simulink model "SecRwRtStHdrstFwdBkwdCtrl"  (R2018b)
settings: Solver=FixedStepDiscrete  StartTime=0.0  StopTime=10.0  FixedStep=0.01  RelTol=1e-3
undefined symbols (not defined in the file or in its folder): KeSMSuMdMotFinshdTm_Val, KeSMSuMdRetryTm1_Val, KeSMSuModeReqDurgTm_Val, KeSMSwSecRwRtStHdrstFwdBkwdEnTrigBitMask_Val
libraries: StCtrlLib x1
settings Model: Creator=sn2xws  LastModifiedBy=sn2xws
settings DataIOCC: SaveFormat=StructureWithTime
settings OptimizationCC: DefaultParameterBehavior=Inlined  EnhancedBackFolding=on  PassReuseOutputArgsAs=Individual arguments  ZeroExternalMemoryAtStartup=off  ZeroInternalMemoryAtStartup=off  OptimizeBlockOrder=speed  DifferentSizesBufferReuse=on  OptimizationCustomize=off
settings DebuggingCC: ParameterTunabilityLossMsg=error
settings ModelReferenceCC: ModelReferenceNumInstancesAllowed=Single
settings SFSimCC: MATLABDynamicMemAlloc=off
settings RTWCC: SystemTargetFile=autosar.tlc  GenCodeOnly=on  TemplateMakefile=ert_default_tmf  Description=AUTOSAR  GenerateReport=on  IncludeHyperlinkInReport=on  LaunchReport=on  GenerateTraceInfo=on  GenerateTraceReport=on  GenerateTraceReportSl=on  GenerateTraceReportSf=on  GenerateTraceReportEml=on
settings CodeAppCC: ForceParamTrailComments=on  IgnoreCustomStorageClasses=off  OperatorAnnotations=on  SimulinkDataObjDesc=on  SFDataObjDesc=on  InsertBlockDesc=on
settings STFCustomTargetCC: TargetLangStandard=C99 (ISO)  MultiwordLength=256  ParMdlRefBuildCompliant=on  CompOptLevelCompliant=on  IncludeMdlTerminateFcn=off  CombineOutputUpdateFcns=on  SuppressErrorStatus=on  ERTCustomFileBanners=on  SupportNonFinite=off  SupportComplex=off  SupportContinuousTime=off  SupportNonInlinedSFcns=off  RemoveResetFunc=on  MATLABClassNameForMDSCustomization=Simulink.SoftwareTarget.ERTCustomization  AutosarCompliant=on  UseToolchainInfoCompliant=on  LookupTableObjectStructAxisOrder=2,1,3,4,...  LUTObjectStructOrderEvenSpacing=Size,Table,Breakpoints  SystemTargetFile=autosar.tlc
settings ERTTargetCC: TargetLangStandard=C99 (ISO)  ConcurrentExecutionCompliant=off  IncludeMdlTerminateFcn=off  SuppressErrorStatus=on  SupportNonFinite=off  SupportComplex=off  ModelStepFunctionPrototypeControlCompliant=off  CPPClassGenCompliant=off  AutosarCompliant=on  LookupTableObjectStructAxisOrder=2,1,3,4,...  LUTObjectStructOrderEvenSpacing=Size,Table,Breakpoints  InlinedParameterPlacement=NonHierarchical  ERTCustomFileTemplate=example_file_process.tlc  ERTFilePackagingFormat=Compact

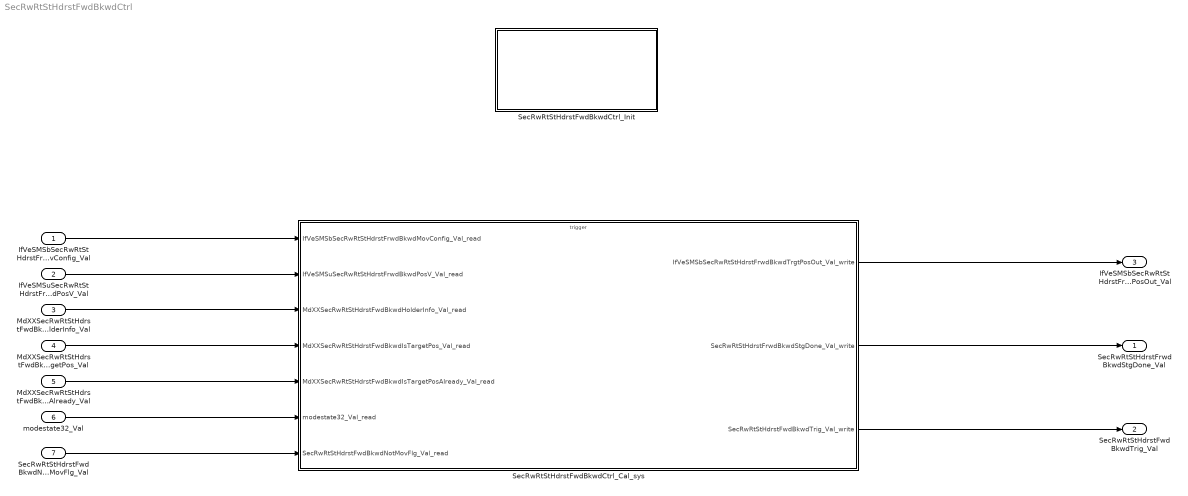
== system SecRwRtStHdrstFwdBkwdCtrl ==
  IfVeSMSbSecRwRtStHdrstFrwdBkwdMovConfig_Val : Inport  OutDataTypeStr=boolean  PortDimensions=1
  IfVeSMSuSecRwRtStHdrstFrwdBkwdPosV_Val : Inport  Port=2  OutDataTypeStr=boolean  PortDimensions=1
  MdXXSecRwRtStHdrstFwdBkwdHolderInfo_Val : Inport  Port=3  OutDataTypeStr=uint32  PortDimensions=1
  MdXXSecRwRtStHdrstFwdBkwdIsTargetPos_Val : Inport  Port=4  OutDataTypeStr=uint32  PortDimensions=1
  MdXXSecRwRtStHdrstFwdBkwdIsTargetPosAlready_Val : Inport  Port=5  OutDataTypeStr=uint32  PortDimensions=1
  modestate32_Val : Inport  Port=6  OutDataTypeStr=uint32  PortDimensions=1
  SecRwRtStHdrstFwdBkwdNotMovFlg_Val : Inport  Port=7  OutDataTypeStr=boolean  PortDimensions=1
  SecRwRtStHdrstFwdBkwdCtrl_Cal_sys : Subsystem
  SecRwRtStHdrstFwdBkwdCtrl_Init : Subsystem
  SecRwRtStHdrstFrwdBkwdStgDone_Val : Outport  OutDataTypeStr=boolean  PortDimensions=1
  SecRwRtStHdrstFwdBkwdTrig_Val : Outport  Port=2  OutDataTypeStr=boolean  PortDimensions=1
  IfVeSMSbSecRwRtStHdrstFrwdBkwdTrgtPosOut_Val : Outport  Port=3  OutDataTypeStr=boolean  PortDimensions=1
  wires:
  IfVeSMSbSecRwRtStHdrstFrwdBkwdMovConfig_Val/1 -> SecRwRtStHdrstFwdBkwdCtrl_Cal_sys/1(IfVeSMSbSecRwRtStHdrstFrwdBkwdMovConfig_Val_read)
  IfVeSMSuSecRwRtStHdrstFrwdBkwdPosV_Val/1 -> SecRwRtStHdrstFwdBkwdCtrl_Cal_sys/2(IfVeSMSuSecRwRtStHdrstFrwdBkwdPosV_Val_read)
  MdXXSecRwRtStHdrstFwdBkwdHolderInfo_Val/1 -> SecRwRtStHdrstFwdBkwdCtrl_Cal_sys/3(MdXXSecRwRtStHdrstFwdBkwdHolderInfo_Val_read)
  MdXXSecRwRtStHdrstFwdBkwdIsTargetPos_Val/1 -> SecRwRtStHdrstFwdBkwdCtrl_Cal_sys/4(MdXXSecRwRtStHdrstFwdBkwdIsTargetPos_Val_read)
  MdXXSecRwRtStHdrstFwdBkwdIsTargetPosAlready_Val/1 -> SecRwRtStHdrstFwdBkwdCtrl_Cal_sys/5(MdXXSecRwRtStHdrstFwdBkwdIsTargetPosAlready_Val_read)
  modestate32_Val/1 -> SecRwRtStHdrstFwdBkwdCtrl_Cal_sys/6(modestate32_Val_read)
  SecRwRtStHdrstFwdBkwdNotMovFlg_Val/1 -> SecRwRtStHdrstFwdBkwdCtrl_Cal_sys/7(SecRwRtStHdrstFwdBkwdNotMovFlg_Val_read)
  SecRwRtStHdrstFwdBkwdCtrl_Cal_sys/1(IfVeSMSbSecRwRtStHdrstFrwdBkwdTrgtPosOut_Val_write) -> IfVeSMSbSecRwRtStHdrstFrwdBkwdTrgtPosOut_Val/1
  SecRwRtStHdrstFwdBkwdCtrl_Cal_sys/2(SecRwRtStHdrstFrwdBkwdStgDone_Val_write) -> SecRwRtStHdrstFrwdBkwdStgDone_Val/1
  SecRwRtStHdrstFwdBkwdCtrl_Cal_sys/3(SecRwRtStHdrstFwdBkwdTrig_Val_write) -> SecRwRtStHdrstFwdBkwdTrig_Val/1

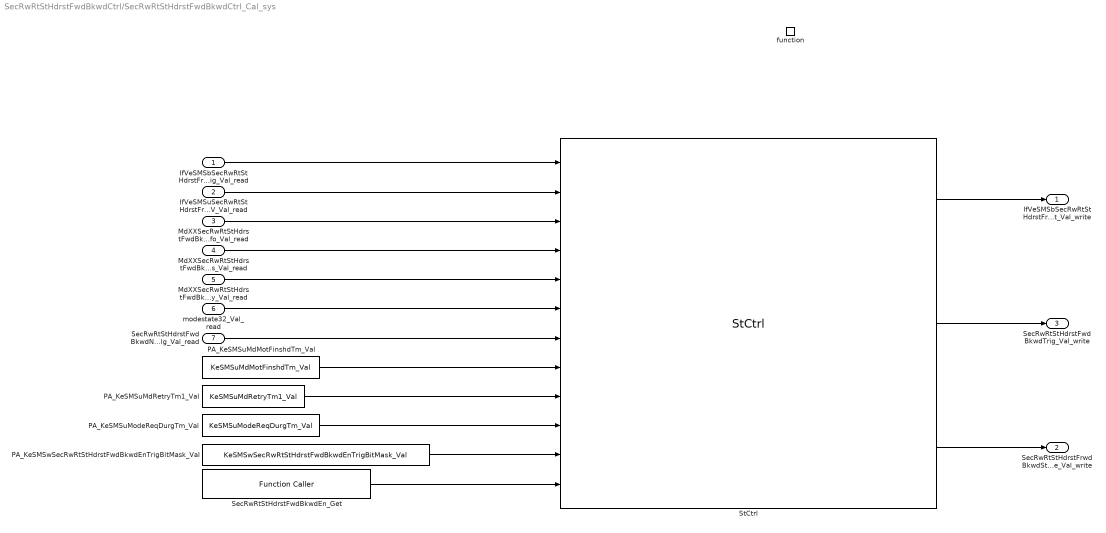
== system SecRwRtStHdrstFwdBkwdCtrl/SecRwRtStHdrstFwdBkwdCtrl_Cal_sys ==
  IfVeSMSbSecRwRtStHdrstFrwdBkwdMovConfig_Val_read : Inport
  IfVeSMSuSecRwRtStHdrstFrwdBkwdPosV_Val_read : Inport  Port=2
  MdXXSecRwRtStHdrstFwdBkwdHolderInfo_Val_read : Inport  Port=3
  MdXXSecRwRtStHdrstFwdBkwdIsTargetPos_Val_read : Inport  Port=4
  MdXXSecRwRtStHdrstFwdBkwdIsTargetPosAlready_Val_read : Inport  Port=5
  modestate32_Val_read : Inport  Port=6
  SecRwRtStHdrstFwdBkwdNotMovFlg_Val_read : Inport  Port=7
  function : TriggerPort  TriggerType=function-call  IsSimulinkFunction=on  FunctionName=SecRwRtStHdrstFwdBkwdCtrl_Cal  VariantControl=(inherit)
  PA_KeSMSuMdMotFinshdTm_Val : Constant  Value=KeSMSuMdMotFinshdTm_Val
  PA_KeSMSuMdRetryTm1_Val : Constant  Value=KeSMSuMdRetryTm1_Val
  PA_KeSMSuModeReqDurgTm_Val : Constant  Value=KeSMSuModeReqDurgTm_Val
  PA_KeSMSwSecRwRtStHdrstFwdBkwdEnTrigBitMask_Val : Constant  Value=KeSMSwSecRwRtStHdrstFwdBkwdEnTrigBitMask_Val
  SecRwRtStHdrstFwdBkwdEn_Get : FunctionCaller  FunctionPrototype=data = SecRwRtStHdrstFwdBkwdEn_Get()  OutputArgumentSpecifications=uint32(1)
  StCtrl : StCtrlLib/StCtrl  SystemSampleTime=-1
  IfVeSMSbSecRwRtStHdrstFrwdBkwdTrgtPosOut_Val_write : Outport
      settings: EnsureOutportIsVirtual=on
  SecRwRtStHdrstFrwdBkwdStgDone_Val_write : Outport  Port=2
      settings: EnsureOutportIsVirtual=on
  SecRwRtStHdrstFwdBkwdTrig_Val_write : Outport  Port=3
      settings: EnsureOutportIsVirtual=on
  wires:
  PA_KeSMSwSecRwRtStHdrstFwdBkwdEnTrigBitMask_Val/1 -> StCtrl/11
  SecRwRtStHdrstFwdBkwdEn_Get/1 -> StCtrl/12
  PA_KeSMSuMdMotFinshdTm_Val/1 -> StCtrl/8
  PA_KeSMSuModeReqDurgTm_Val/1 -> StCtrl/10
  PA_KeSMSuMdRetryTm1_Val/1 -> StCtrl/9
  IfVeSMSbSecRwRtStHdrstFrwdBkwdMovConfig_Val_read/1 -> StCtrl/1
  IfVeSMSuSecRwRtStHdrstFrwdBkwdPosV_Val_read/1 -> StCtrl/2
  MdXXSecRwRtStHdrstFwdBkwdHolderInfo_Val_read/1 -> StCtrl/3
  MdXXSecRwRtStHdrstFwdBkwdIsTargetPos_Val_read/1 -> StCtrl/4
  MdXXSecRwRtStHdrstFwdBkwdIsTargetPosAlready_Val_read/1 -> StCtrl/5
  modestate32_Val_read/1 -> StCtrl/6
  SecRwRtStHdrstFwdBkwdNotMovFlg_Val_read/1 -> StCtrl/7
  StCtrl/1 -> IfVeSMSbSecRwRtStHdrstFrwdBkwdTrgtPosOut_Val_write/1
  StCtrl/2 -> SecRwRtStHdrstFwdBkwdTrig_Val_write/1
  StCtrl/3 -> SecRwRtStHdrstFrwdBkwdStgDone_Val_write/1

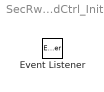
== system SecRwRtStHdrstFwdBkwdCtrl/SecRwRtStHdrstFwdBkwdCtrl_Init ==
  Event Listener : EventListener  EventName=reset
